simulink model "friction_rt_online"  (R2025a)
settings: Solver=VariableStepAuto  StartTime=0.0  StopTime=10  RelTol=1e-3
settings Model: Creator=Kylo_Ren  LastModifiedBy=Kylo_Ren

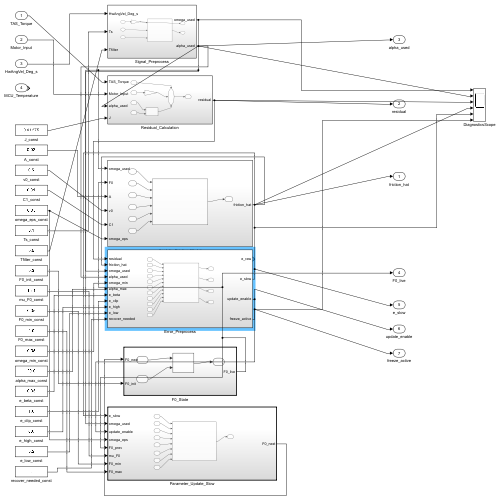
[thumbnail: Simulink's stored preview of the top-level diagram]
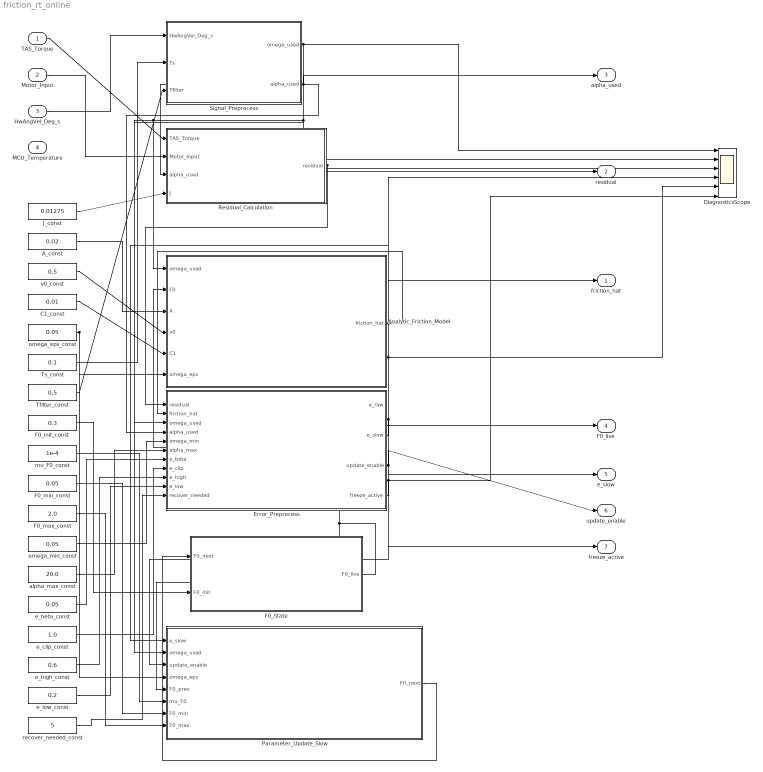
== system friction_rt_online ==
  TAS_Torque : Inport
  Motor_Input : Inport  Port=2
  HwAngVel_Deg_s : Inport  Port=3
  MCU_Temperature : Inport  Port=4
  A_const : Constant  Value=0.02
  Analytic_Friction_Model : Subsystem
  C1_const : Constant  Value=0.01
  DiagnosticsScope : Scope  NumInputPorts=6
  Error_Preprocess : Subsystem
  F0_State : Subsystem  TreatAsAtomicUnit=on
  F0_init_const : Constant  Value=0.3
  F0_max_const : Constant  Value=2.0
  F0_min_const : Constant  Value=0.05
  J_const : Constant  Value=0.01275
  Parameter_Update_Slow : Subsystem  TreatAsAtomicUnit=on
  Residual_Calculation : Subsystem
  Signal_Preprocess : Subsystem
  Tfilter_const : Constant  Value=0.5
  Ts_const : Constant  Value=0.1
  alpha_max_const : Constant  Value=20.0
  e_beta_const : Constant  Value=0.05
  e_clip_const : Constant  Value=1.0
  e_high_const : Constant  Value=0.6
  e_low_const : Constant  Value=0.2
  mu_F0_const : Constant  Value=1e-4
  omega_eps_const : Constant  Value=0.05
  omega_min_const : Constant  Value=0.05
  recover_needed_const : Constant  Value=5
  v0_const : Constant  Value=0.5
  friction_hat : Outport
  residual : Outport  Port=2
  alpha_used : Outport  Port=3
  F0_live : Outport  Port=4
  e_slow : Outport  Port=5
  update_enable : Outport  Port=6
  freeze_active : Outport  Port=7
  wires:
  HwAngVel_Deg_s/1 -> Signal_Preprocess/1(HwAngVel_Deg_s)
  Ts_const/1 -> Signal_Preprocess/2(Ts)
  Tfilter_const/1 -> Signal_Preprocess/3(Tfilter)
  Signal_Preprocess/1(omega_used) -> Analytic_Friction_Model/1(omega_used), Parameter_Update_Slow/2(omega_used), Error_Preprocess/3(omega_used), DiagnosticsScope/1
  Signal_Preprocess/2(alpha_used) -> Residual_Calculation/3(alpha_used), Error_Preprocess/4(alpha_used), alpha_used/1, DiagnosticsScope/2
  TAS_Torque/1 -> Residual_Calculation/1(TAS_Torque)
  Motor_Input/1 -> Residual_Calculation/2(Motor_Input)
  J_const/1 -> Residual_Calculation/4(J)
  Residual_Calculation/1(residual) -> Error_Preprocess/1(residual), residual/1, DiagnosticsScope/3
  Analytic_Friction_Model/1(friction_hat) -> Error_Preprocess/2(friction_hat), friction_hat/1, DiagnosticsScope/4
  omega_min_const/1 -> Error_Preprocess/5(omega_min)
  alpha_max_const/1 -> Error_Preprocess/6(alpha_max)
  e_beta_const/1 -> Error_Preprocess/7(e_beta)
  e_clip_const/1 -> Error_Preprocess/8(e_clip)
  e_high_const/1 -> Error_Preprocess/9(e_high)
  e_low_const/1 -> Error_Preprocess/10(e_low)
  recover_needed_const/1 -> Error_Preprocess/11(recover_needed)
  Error_Preprocess/2(e_slow) -> Parameter_Update_Slow/1(e_slow), DiagnosticsScope/5, e_slow/1
  Error_Preprocess/3(update_enable) -> update_enable/1, Parameter_Update_Slow/3(update_enable)
  omega_eps_const/1 -> Parameter_Update_Slow/4(omega_eps), Analytic_Friction_Model/6(omega_eps)
  F0_State/1(F0_live) -> Analytic_Friction_Model/2(F0), F0_live/1, Parameter_Update_Slow/5(F0_prev)
  mu_F0_const/1 -> Parameter_Update_Slow/6(mu_F0)
  F0_min_const/1 -> Parameter_Update_Slow/7(F0_min)
  F0_max_const/1 -> Parameter_Update_Slow/8(F0_max)
  Parameter_Update_Slow/1(F0_next) -> F0_State/1(F0_next)
  F0_init_const/1 -> F0_State/2(F0_init)
  A_const/1 -> Analytic_Friction_Model/3(A)
  v0_const/1 -> Analytic_Friction_Model/4(v0)
  C1_const/1 -> Analytic_Friction_Model/5(C1)
  Error_Preprocess/4(freeze_active) -> freeze_active/1, DiagnosticsScope/6

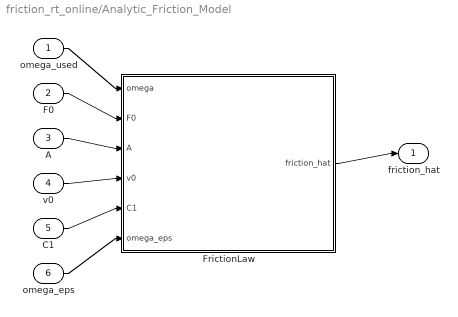
== system friction_rt_online/Analytic_Friction_Model ==
  omega_used : Inport
  F0 : Inport  Port=2
  A : Inport  Port=3
  v0 : Inport  Port=4
  C1 : Inport  Port=5
  omega_eps : Inport  Port=6
  FrictionLaw : MATLAB Function  TreatAsAtomicUnit=on
  friction_hat : Outport
  wires:
  omega_used/1 -> FrictionLaw/1(omega)
  F0/1 -> FrictionLaw/2(F0)
  A/1 -> FrictionLaw/3(A)
  v0/1 -> FrictionLaw/4(v0)
  C1/1 -> FrictionLaw/5(C1)
  omega_eps/1 -> FrictionLaw/6(omega_eps)
  FrictionLaw/1(friction_hat) -> friction_hat/1

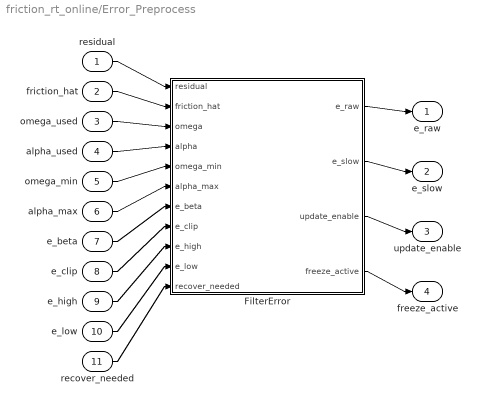
== system friction_rt_online/Error_Preprocess ==
  residual : Inport
  friction_hat : Inport  Port=2
  omega_used : Inport  Port=3
  alpha_used : Inport  Port=4
  omega_min : Inport  Port=5
  alpha_max : Inport  Port=6
  e_beta : Inport  Port=7
  e_clip : Inport  Port=8
  e_high : Inport  Port=9
  e_low : Inport  Port=10
  recover_needed : Inport  Port=11
  FilterError : MATLAB Function  TreatAsAtomicUnit=on
  e_raw : Outport
  e_slow : Outport  Port=2
  update_enable : Outport  Port=3
  freeze_active : Outport  Port=4
  wires:
  residual/1 -> FilterError/1(residual)
  friction_hat/1 -> FilterError/2(friction_hat)
  omega_used/1 -> FilterError/3(omega)
  alpha_used/1 -> FilterError/4(alpha)
  omega_min/1 -> FilterError/5(omega_min)
  alpha_max/1 -> FilterError/6(alpha_max)
  e_beta/1 -> FilterError/7(e_beta)
  e_clip/1 -> FilterError/8(e_clip)
  e_high/1 -> FilterError/9(e_high)
  e_low/1 -> FilterError/10(e_low)
  recover_needed/1 -> FilterError/11(recover_needed)
  FilterError/1(e_raw) -> e_raw/1
  FilterError/2(e_slow) -> e_slow/1
  FilterError/3(update_enable) -> update_enable/1
  FilterError/4(freeze_active) -> freeze_active/1

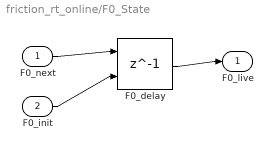
== system friction_rt_online/F0_State ==
  F0_next : Inport
  F0_init : Inport  Port=2
  F0_delay : Delay  DelayLength=1  InitialConditionSource=Input port
      settings: InputPortMap=u0,p4
  F0_live : Outport
  wires:
  F0_next/1 -> F0_delay/1
  F0_init/1 -> F0_delay/2
  F0_delay/1 -> F0_live/1

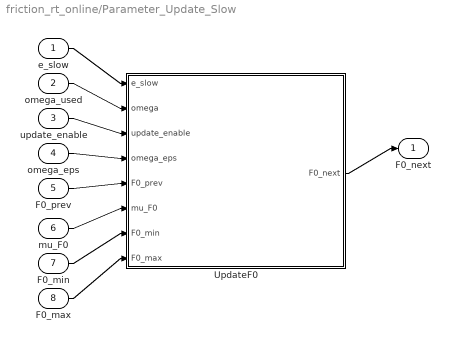
== system friction_rt_online/Parameter_Update_Slow ==
  e_slow : Inport
  omega_used : Inport  Port=2
  update_enable : Inport  Port=3
  omega_eps : Inport  Port=4
  F0_prev : Inport  Port=5
  mu_F0 : Inport  Port=6
  F0_min : Inport  Port=7
  F0_max : Inport  Port=8
  UpdateF0 : MATLAB Function  TreatAsAtomicUnit=on
  F0_next : Outport
  wires:
  e_slow/1 -> UpdateF0/1(e_slow)
  omega_used/1 -> UpdateF0/2(omega)
  update_enable/1 -> UpdateF0/3(update_enable)
  omega_eps/1 -> UpdateF0/4(omega_eps)
  F0_prev/1 -> UpdateF0/5(F0_prev)
  mu_F0/1 -> UpdateF0/6(mu_F0)
  F0_min/1 -> UpdateF0/7(F0_min)
  F0_max/1 -> UpdateF0/8(F0_max)
  UpdateF0/1(F0_next) -> F0_next/1

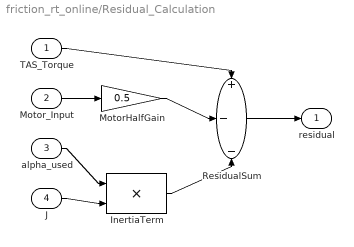
== system friction_rt_online/Residual_Calculation ==
  TAS_Torque : Inport
  Motor_Input : Inport  Port=2
  alpha_used : Inport  Port=3
  J : Inport  Port=4
  InertiaTerm : Product
  MotorHalfGain : Gain  Gain=0.5
  ResidualSum : Sum  Inputs=+--
  residual : Outport
  wires:
  TAS_Torque/1 -> ResidualSum/1
  Motor_Input/1 -> MotorHalfGain/1
  MotorHalfGain/1 -> ResidualSum/2
  alpha_used/1 -> InertiaTerm/1
  J/1 -> InertiaTerm/2
  InertiaTerm/1 -> ResidualSum/3
  ResidualSum/1 -> residual/1

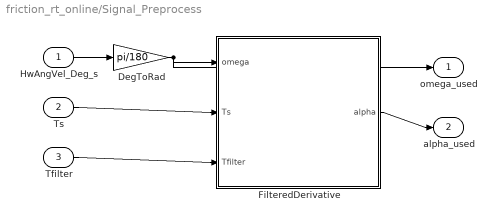
== system friction_rt_online/Signal_Preprocess ==
  HwAngVel_Deg_s : Inport
  Ts : Inport  Port=2
  Tfilter : Inport  Port=3
  DegToRad : Gain  Gain=pi/180
  FilteredDerivative : MATLAB Function  TreatAsAtomicUnit=on
  omega_used : Outport
  alpha_used : Outport  Port=2
  wires:
  HwAngVel_Deg_s/1 -> DegToRad/1
  DegToRad/1 -> FilteredDerivative/1(omega), omega_used/1
  Ts/1 -> FilteredDerivative/2(Ts)
  Tfilter/1 -> FilteredDerivative/3(Tfilter)
  FilteredDerivative/1(alpha) -> alpha_used/1

== matlab function friction_rt_online/Analytic_Friction_Model/FrictionLaw ==
  data: omega input; friction_hat output; F0 input; A input; v0 input; C1 input; omega_eps input
function friction_hat = fcn(omega, F0, A, v0, C1, omega_eps)                             
                                                                                        % Analytic friction law:                                                                 
                                                                                        % friction_hat = tanh(omega/omega_eps) * (F0 + A*(1-exp(-abs(omega)/v0)) + C1*abs(omega))
                                                                                        absw = abs(omega);                                                                       
                                                                                        s = tanh(omega / max(omega_eps, 1e-6));                                                  
                                                                                        phi = 1.0 - exp(-absw / max(v0, 1e-6));                                                  
                                                                                        mag = F0 + A * phi + C1 * absw;                                                          
                                                                                        if mag < 0.0                                                                             
                                                                                            mag = 0.0;                                                                           
                                                                                        end                                                                                      
                                                                                        friction_hat = s * mag;

== matlab function friction_rt_online/Signal_Preprocess/FilteredDerivative ==
  data: omega input; alpha output; Ts input; Tfilter input
function alpha = fcn(omega, Ts, Tfilter)        
                                               % Filtered derivative used for the inertia term.
                                               % X[k] = (Ts/T) * omega[k] + (1 - Ts/T) * X[k-1]
                                               % alpha[k] = (1/T) * (omega[k] - X[k-1])        
                                               persistent x_prev                               
                                               if isempty(x_prev)                              
                                                   x_prev = omega;                             
                                               end                                             
                                               a = Ts / max(Tfilter, 1e-6);                    
                                               a = min(max(a, 0.0), 1.0);                      
                                               alpha = (omega - x_prev) / max(Tfilter, 1e-6);  
                                               x_new = a * omega + (1.0 - a) * x_prev;         
                                               x_prev = x_new;

== matlab function friction_rt_online/Error_Preprocess/FilterError ==
  data: residual input; e_raw output; friction_hat input; omega input; alpha input; omega_min input; alpha_max input; e_beta input; e_clip input; e_high input; e_low input; recover_needed input; e_slow output; update_enable output; freeze_active output
function [e_raw, e_slow, update_enable, freeze_active] = fcn(residual, friction_hat, omega, alpha, omega_min, alpha_max, e_beta, e_clip, e_high, e_low, recover_needed)
  % Build a reliable adaptation error.                                                                                                                                   
  % Enter freeze on anomaly; exit freeze only after recovery is sustained.                                                                                               
  persistent e_prev freeze_state recover_count                                                                                                                           
  if isempty(e_prev)                                                                                                                                                     
      e_prev = 0.0;                                                                                                                                                      
      freeze_state = false;                                                                                                                                              
      recover_count = 0;                                                                                                                                                 
  end                                                                                                                                                                    
  e_raw = residual - friction_hat;                                                                                                                                       
  trusted_sample = (abs(omega) > omega_min) && (abs(alpha) < alpha_max);                                                                                                 
  anomaly = (abs(e_raw) > e_high) || (abs(alpha) > alpha_max);                                                                                                           
  recovered = trusted_sample && (abs(e_raw) < e_low);                                                                                                                    
  if ~freeze_state && anomaly                                                                                                                                            
      freeze_state = true;                                                                                                                                               
      recover_count = 0;                                                                                                                                                 
  elseif freeze_state                                                                                                                                                    
      if recovered                                                                                                                                                       
          recover_count = recover_count + 1;                                                                                                                             
          if recover_count >= recover_needed                                                                                                                             
              freeze_state = false;                                                                                                                                      
              recover_count = 0;                                                                                                                                         
          end                                                                                                                                                            
      else                                                                                                                                                               
          recover_count = 0;                                                                                                                                             
      end                                                                                                                                                                
  end                                                                                                                                                                    
  freeze_active = freeze_state;                                                                                                                                          
  update_enable = trusted_sample && ~freeze_state;                                                                                                                       
  e_used = e_raw;                                                                                                                                                        
  if e_used > e_clip                                                                                                                                                     
      e_used = e_clip;                                                                                                                                                   
  elseif e_used < -e_clip                                                                                                                                                
      e_used = -e_clip;                                                                                                                                                  
  end                                                                                                                                                                    
  if update_enable                                                                                                                                                       
      beta = min(max(e_beta, 0.0), 1.0);                                                                                                                                 
      e_prev = (1.0 - beta) * e_prev + beta * e_used;                                                                                                                    
  end                                                                                                                                                                    
  e_slow = e_prev;

== matlab function friction_rt_online/Parameter_Update_Slow/UpdateF0 ==
  data: e_slow input; F0_next output; omega input; update_enable input; omega_eps input; F0_prev input; mu_F0 input; F0_min input; F0_max input
function F0_next = fcn(e_slow, omega, update_enable, omega_eps, F0_prev, mu_F0, F0_min, F0_max)
                                                                                              % Slow F0 adaptation using a filtered error instead of raw instantaneous residual.             
                                                                                              s = tanh(omega / max(omega_eps, 1e-6));                                                        
                                                                                              F0_next = F0_prev;                                                                             
                                                                                              if update_enable                                                                               
                                                                                                  F0_next = F0_prev + mu_F0 * e_slow * s;                                                    
                                                                                              end                                                                                            
                                                                                              if F0_next < F0_min                                                                            
                                                                                                  F0_next = F0_min;                                                                          
                                                                                              elseif F0_next > F0_max                                                                        
                                                                                                  F0_next = F0_max;                                                                          
                                                                                              end
